simulink model "UAVFeedbackLinearize"  (R2023a)
settings: Solver=ode45  StartTime=0.0  StopTime=12  RelTol=1e-3  EnableMultiTasking=on
settings Model: Creator=user  LastModifiedBy=weetsj
settings SolverCC: AlgebraicLoopSolver=TrustRegion
settings DataIOCC: LimitDataPoints=on  SaveFormat=Array  ReturnWorkspaceOutputs=off
settings OptimizationCC: LifeSpan=inf
settings DebuggingCC: UnconnectedInputMsg=warning  UnconnectedOutputMsg=warning  UnconnectedLineMsg=warning  SFUnexpectedBacktrackingDiag=warning  SFNoUnconditionalDefaultTransitionDiag=warning  SFExecutionAtInitializationDiag=none  ArithmeticOperatorsInVariantConditions=warning
settings HardwareCC: ProdBitPerPointer=32  ProdBitPerSizeT=32  ProdBitPerPtrDiffT=32  ProdLargestAtomicFloat=None  ProdIntDivRoundTo=Undefined  ProdEndianess=Unspecified  ProdWordSize=32  ProdHWDeviceType=32-bit Generic
settings ModelReferenceCC: EnableRefExpFcnMdlSchedulingChecks=on  PropagateSignalLabelsOutOfModel=off
settings SFSimCC: SimUseLocalCustomCode=off  CustomCodeUndefinedFunction=UseInterfaceOnly
settings RTWCC: RTWUseLocalCustomCode=off
settings CodeAppCC: StateflowObjectComments=on
settings GRTTargetCC: TargetLangStandard=C89/C90 (ANSI)
settings ConfigComp: CovMetricSettings=dw  CovSaveCumulativeToWorkspaceVar=on  CovSaveSingleToWorkspaceVar=on  CovExternalEMLEnable=off

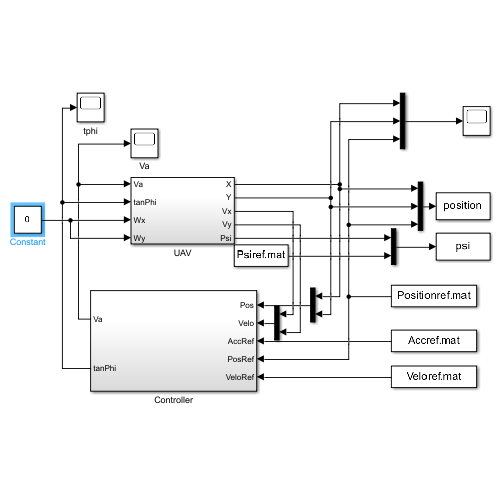
[thumbnail: Simulink's stored preview of the top-level diagram]
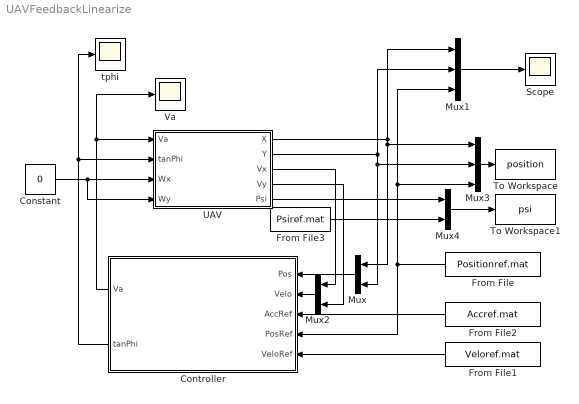
== system UAVFeedbackLinearize ==
  Constant : Constant  Value=0
  Controller : Subsystem
  From File : FromFile  FileName=Positionref.mat  SampleTime=0
  From File1 : FromFile  FileName=Veloref.mat  SampleTime=0
  From File2 : FromFile  FileName=Accref.mat  SampleTime=0
  From File3 : FromFile  FileName=Psiref.mat  SampleTime=0
  Mux : Mux  Inputs=2
  Mux1 : Mux  Inputs=3
  Mux2 : Mux  Inputs=2
  Mux3 : Mux  Inputs=3
  Mux4 : Mux  Inputs=2
  Scope : Scope
  To Workspace : ToWorkspace  VariableName=position  SaveFormat=Structure With Time  SampleTime=-1
  To Workspace1 : ToWorkspace  VariableName=psi  SaveFormat=Structure With Time  SampleTime=-1
  UAV : Subsystem
  Va : Scope
  tphi : Scope
  wires:
  From File2/1 -> Controller/3(AccRef)
  From File1/1 -> Controller/5(VeloRef)
  Mux/1 -> Controller/1(Pos)
  Controller/1(Va) -> Va/1, UAV/1(Va)
  Controller/2(tanPhi) -> tphi/1, UAV/2(tanPhi)
  Constant/1 -> UAV/4(Wy), UAV/3(Wx)
  Mux1/1 -> Scope/1
  UAV/1(X) -> Mux/1, Mux3/1, Mux1/1
  UAV/2(Y) -> Mux3/2, Mux/2, Mux1/2
  From File/1 -> Mux3/3, Mux1/3, Controller/4(PosRef)
  Mux2/1 -> Controller/2(Velo)
  UAV/3(Vx) -> Mux2/1
  UAV/4(Vy) -> Mux2/2
  Mux3/1 -> To Workspace/1
  UAV/5(Psi) -> Mux4/1
  Mux4/1 -> To Workspace1/1
  From File3/1 -> Mux4/2

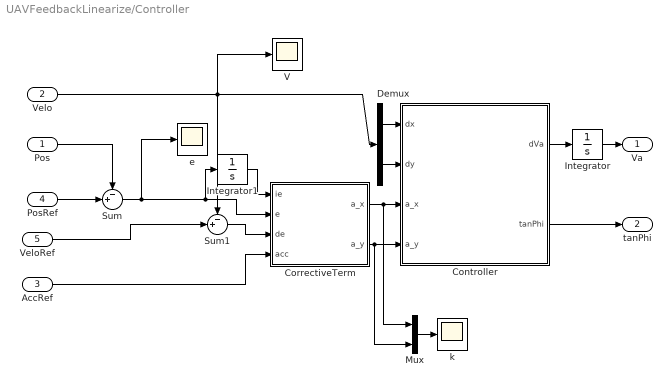
== system UAVFeedbackLinearize/Controller ==
  Pos : Inport
  Velo : Inport  Port=2
  AccRef : Inport  Port=3
  PosRef : Inport  Port=4
  VeloRef : Inport  Port=5
  Controller : MATLAB Function  TreatAsAtomicUnit=on
  CorrectiveTerm : MATLAB Function  TreatAsAtomicUnit=on
  Demux : Demux  Outputs=2
  Integrator : Integrator  InitialCondition=20
  Integrator1 : Integrator  InitialCondition=20
  Mux : Mux  Inputs=2
  Sum : Sum  Inputs=-+|
  Sum1 : Sum  Inputs=-+|
  V : Scope
  e : Scope
  k : Scope
  Va : Outport  VectorParamsAs1DForOutWhenUnconnected=off
  tanPhi : Outport  Port=2  VectorParamsAs1DForOutWhenUnconnected=off
  wires:
  Controller/2(tanPhi) -> tanPhi/1
  PosRef/1 -> Sum/2
  Pos/1 -> Sum/1
  VeloRef/1 -> Sum1/2
  CorrectiveTerm/1(a_x) -> Mux/1, Controller/3(a_x)
  CorrectiveTerm/2(a_y) -> Mux/2, Controller/4(a_y)
  Sum1/1 -> CorrectiveTerm/3(de)
  Sum/1 -> e/1, Integrator1/1, CorrectiveTerm/2(e)
  AccRef/1 -> CorrectiveTerm/4(acc)
  Demux/1 -> Controller/1(dx)
  Demux/2 -> Controller/2(dy)
  Controller/1(dVa) -> Integrator/1
  Integrator/1 -> Va/1
  Velo/1 -> V/1, Demux/1, Sum1/1
  Mux/1 -> k/1
  Integrator1/1 -> CorrectiveTerm/1(ie)

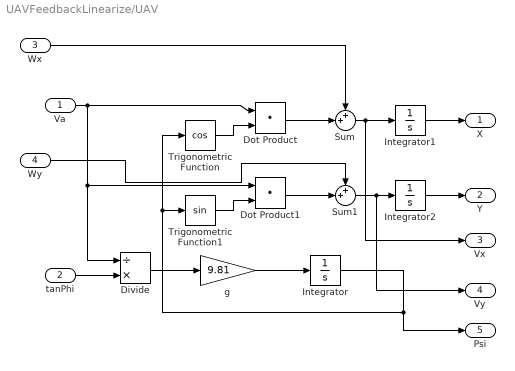
== system UAVFeedbackLinearize/UAV ==
  Va : Inport
  tanPhi : Inport  Port=2
  Wx : Inport  Port=3
  Wy : Inport  Port=4
  Divide : Product  Inputs=/*
  Dot Product : DotProduct  OutDataTypeStr=Inherit: Inherit via internal rule
  Dot Product1 : DotProduct  OutDataTypeStr=Inherit: Inherit via internal rule
  Integrator : Integrator
  Integrator1 : Integrator
  Integrator2 : Integrator
  Sum : Sum  Inputs=++|
  Sum1 : Sum  Inputs=++|
  Trigonometric Function : Trigonometry  Operator=cos
  Trigonometric Function1 : Trigonometry
  g : Gain  Gain=9.81
  X : Outport  VectorParamsAs1DForOutWhenUnconnected=off
  Y : Outport  Port=2  VectorParamsAs1DForOutWhenUnconnected=off
  Vx : Outport  Port=3  VectorParamsAs1DForOutWhenUnconnected=off
  Vy : Outport  Port=4  VectorParamsAs1DForOutWhenUnconnected=off
  Psi : Outport  Port=5  VectorParamsAs1DForOutWhenUnconnected=off
  wires:
  tanPhi/1 -> Divide/2
  Divide/1 -> g/1
  g/1 -> Integrator/1
  Integrator/1 -> Trigonometric Function1/1, Trigonometric Function/1, Psi/1
  Trigonometric Function/1 -> Dot Product/2
  Va/1 -> Dot Product1/1, Divide/1, Dot Product/1
  Trigonometric Function1/1 -> Dot Product1/2
  Integrator1/1 -> X/1
  Integrator2/1 -> Y/1
  Dot Product/1 -> Sum/2
  Sum/1 -> Vx/1, Integrator1/1
  Wx/1 -> Sum/1
  Dot Product1/1 -> Sum1/2
  Sum1/1 -> Vy/1, Integrator2/1
  Wy/1 -> Sum1/1

== matlab function UAVFeedbackLinearize/Controller/CorrectiveTerm ==
  data: ie input; e input; a_x output; de input; acc input; a_y output
function [a_x,a_y] = fcn(ie, e,de,acc)
%#codegen
Kp=[3 3];
Kd=[3 3];
Ki=[1 1];
k=acc+Kp*e+Kd*de + Ki*ie;
a_x=k(1);a_y=k(2);

== matlab function UAVFeedbackLinearize/Controller/Controller ==
  data: dVa output; dx input; tanPhi output; dy input; a_x input; a_y input
function [dVa,tanPhi] = fcn(dx,dy,a_x,a_y)
%#codegen
g=9.81;
tanPhi=1/g*(-a_x*dy+a_y*dx)/sqrt(dx^2+dy^2);
dVa=(a_x*dx+a_y*dy)/sqrt(dx^2+dy^2);
